simulink model "Q4EQ1"  (R2026a)
settings: Solver=VariableStepAuto

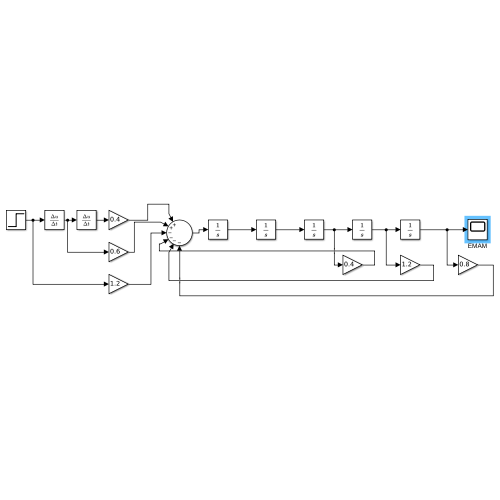
[thumbnail: Simulink's stored preview of the top-level diagram]
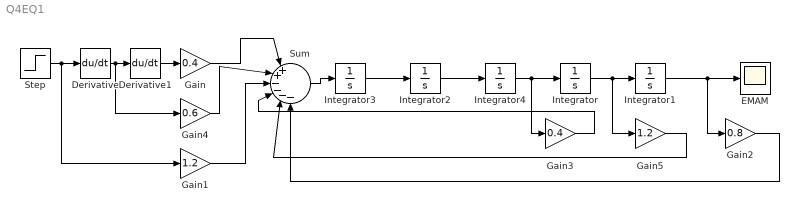
== system Q4EQ1 ==
  Derivative : Derivative
  Derivative1 : Derivative
  EMAM : Scope
      settings: ActiveDisplayYMinimum=-5.363470445318724E+15  ActiveDisplayYMaximum=2.8047808752891548E+16
  Gain : Gain  Gain=0.4
  Gain1 : Gain  Gain=1.2
  Gain2 : Gain  Gain=0.8
  Gain3 : Gain  Gain=0.4
  Gain4 : Gain  Gain=0.6
  Gain5 : Gain  Gain=1.2
  Integrator{,1..4} (5 alike) : Integrator
  Step : Step  SampleTime=0
  Sum : Sum  Inputs=|++----
  wires:
  Step/1 -> Gain1/1, Derivative/1
  Gain/1 -> Sum/1
  Gain4/1 -> Sum/2
  Sum/1 -> Integrator3/1
  Integrator3/1 -> Integrator2/1
  Integrator2/1 -> Integrator4/1
  Integrator4/1 -> Gain3/1, Integrator/1
  Integrator/1 -> Gain5/1, Integrator1/1
  Integrator1/1 -> EMAM/1, Gain2/1
  Derivative/1 -> Gain4/1, Derivative1/1
  Derivative1/1 -> Gain/1
  Gain1/1 -> Sum/3
  Gain3/1 -> Sum/4
  Gain5/1 -> Sum/5
  Gain2/1 -> Sum/6
